simulink model "Q2_2"  (R2016a)
settings: Solver=VariableStepAuto  StartTime=0.0  StopTime=10.0  RelTol=1e-3
values from neighbouring files (symbols this model uses):
  c = -M*l^2 * Theta(1)    [Q2_3.m]
  g = 9.81    [Q2_3.m]
  l = -g/Theta(2)    [Q2_3.m]
undefined symbols (not defined in the file or in its folder): theta_pend
settings Model: Creator=masom  LastModifiedBy=masom

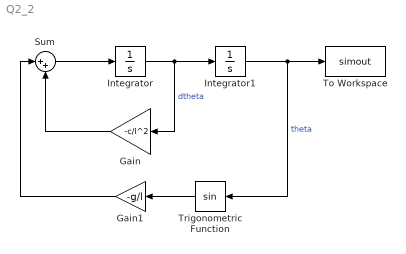
== system Q2_2 ==
  Gain : Gain  Gain=-c/l^2
  Gain1 : Gain  Gain=-g/l
  Integrator : Integrator
  Integrator1 : Integrator  InitialCondition=theta_pend(4)
  Sum : Sum  Inputs=|++
  To Workspace : ToWorkspace  VariableName=simout  SaveFormat=Timeseries  SampleTime=-1
  Trigonometric Function : Trigonometry
  wires:
  Integrator/1 -> Gain/1, Integrator1/1  "dtheta"
  Integrator1/1 -> Trigonometric Function/1, To Workspace/1  "theta"
  Sum/1 -> Integrator/1
  Gain/1 -> Sum/2
  Gain1/1 -> Sum/1
  Trigonometric Function/1 -> Gain1/1
